simulink model "M1_P2"  (R2023a)
settings: Solver=VariableStepAuto  StartTime=0.0  StopTime=0.35  RelTol=1e-3
undefined symbols (not defined in the file): f_eff, J_eff, Kb, Ktn, L, R
settings Model: Creator=azzam  LastModifiedBy=azzam

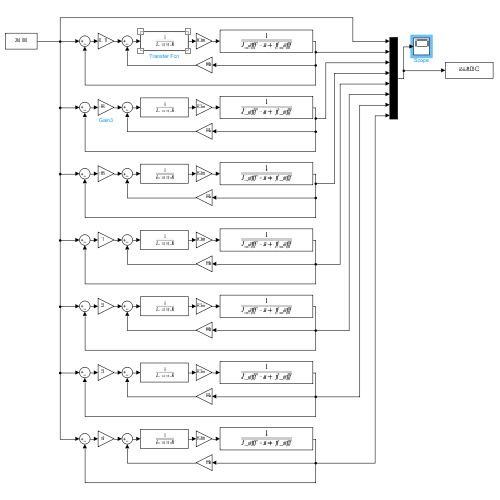
[thumbnail: Simulink's stored preview of the top-level diagram]
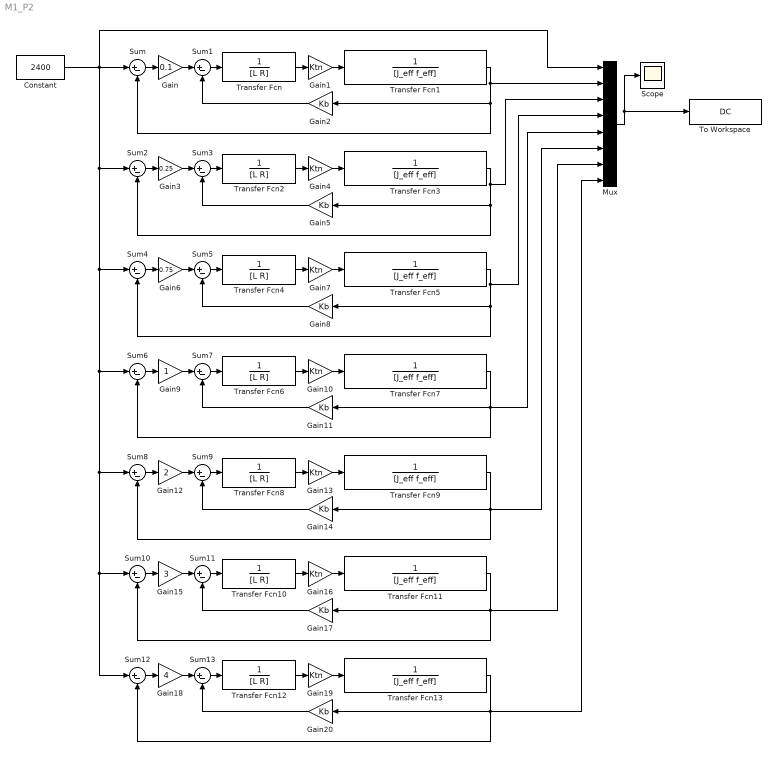
== system M1_P2 ==
  Constant : Constant  Value=2400
  Gain : Gain  Gain=0.1
  Gain{1,4,7,10,13,16,19} (7 alike) : Gain  Gain=Ktn
  Gain{2,5,8,11,14,17,20} (7 alike) : Gain  Gain=Kb
  Gain12 : Gain  Gain=2
  Gain15 : Gain  Gain=3
  Gain18 : Gain  Gain=4
  Gain3 : Gain  Gain=0.25
  Gain6 : Gain  Gain=0.75
  Gain9 : Gain
  Mux : Mux  Inputs=8
  Scope : Scope
  Sum{,1..13} (14 alike) : Sum  Inputs=|+-
  To Workspace : ToWorkspace  VariableName=DC  SaveFormat=Timeseries  SampleTime=-1
  Transfer Fcn{,2,4,6,8,10,12} (7 alike) : TransferFcn  Denominator=[L R]
  Transfer Fcn{1,3,5,7,9,11,13} (7 alike) : TransferFcn  Denominator=[J_eff f_eff]
  wires:
  Sum/1 -> Gain/1
  Gain/1 -> Sum1/1
  Sum1/1 -> Transfer Fcn/1
  Transfer Fcn/1 -> Gain1/1
  Gain1/1 -> Transfer Fcn1/1
  Gain2/1 -> Sum1/2
  Constant/1 -> Mux/1, Sum12/1, Sum10/1, Sum8/1, Sum6/1, Sum4/1, Sum2/1, Sum/1
  Transfer Fcn1/1 -> Mux/2, Sum/2, Gain2/1
  Mux/1 -> Scope/1, To Workspace/1
  Transfer Fcn3/1 -> Mux/3, Sum2/2, Gain5/1
  Transfer Fcn2/1 -> Gain4/1
  Gain5/1 -> Sum3/2
  Gain3/1 -> Sum3/1
  Sum2/1 -> Gain3/1
  Gain4/1 -> Transfer Fcn3/1
  Sum3/1 -> Transfer Fcn2/1
  Transfer Fcn4/1 -> Gain7/1
  Gain8/1 -> Sum5/2
  Transfer Fcn5/1 -> Mux/4, Sum4/2, Gain8/1
  Gain6/1 -> Sum5/1
  Sum4/1 -> Gain6/1
  Sum5/1 -> Transfer Fcn4/1
  Gain7/1 -> Transfer Fcn5/1
  Transfer Fcn6/1 -> Gain10/1
  Gain11/1 -> Sum7/2
  Transfer Fcn7/1 -> Mux/5, Sum6/2, Gain11/1
  Gain9/1 -> Sum7/1
  Sum6/1 -> Gain9/1
  Sum7/1 -> Transfer Fcn6/1
  Gain10/1 -> Transfer Fcn7/1
  Transfer Fcn8/1 -> Gain13/1
  Gain14/1 -> Sum9/2
  Transfer Fcn9/1 -> Mux/6, Sum8/2, Gain14/1
  Gain12/1 -> Sum9/1
  Sum8/1 -> Gain12/1
  Sum9/1 -> Transfer Fcn8/1
  Gain13/1 -> Transfer Fcn9/1
  Transfer Fcn10/1 -> Gain16/1
  Gain17/1 -> Sum11/2
  Transfer Fcn11/1 -> Mux/7, Sum10/2, Gain17/1
  Gain15/1 -> Sum11/1
  Sum10/1 -> Gain15/1
  Sum11/1 -> Transfer Fcn10/1
  Gain16/1 -> Transfer Fcn11/1
  Transfer Fcn12/1 -> Gain19/1
  Gain20/1 -> Sum13/2
  Transfer Fcn13/1 -> Mux/8, Sum12/2, Gain20/1
  Gain18/1 -> Sum13/1
  Sum12/1 -> Gain18/1
  Sum13/1 -> Transfer Fcn12/1
  Gain19/1 -> Transfer Fcn13/1
